simulink model "lab2"  (R2016a)
settings: Solver=VariableStepAuto  StartTime=0.0  StopTime=100  RelTol=1e-3
settings Model: Creator=ms36124  LastModifiedBy=ms36124

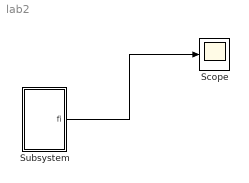
== system lab2 ==
  Scope : Scope
  Subsystem : Subsystem  mask{m=10, k=1, l=3, g=10, fi0=180}
  wires:
  Subsystem/1("fi ") -> Scope/1

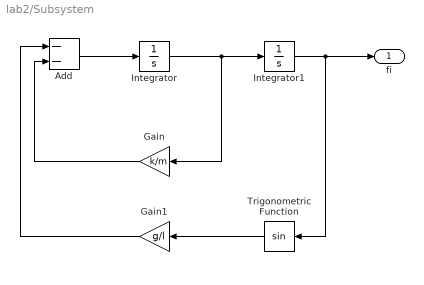
== system lab2/Subsystem ==
  Add : Sum  Inputs=--
  Gain : Gain  Gain=k/m
  Gain1 : Gain  Gain=g/l
  Integrator : Integrator
  Integrator1 : Integrator  InitialCondition=fi0*pi/180
  Trigonometric Function : Trigonometry
  "fi " : Outport
  wires:
  Trigonometric Function/1 -> Gain1/1
  Integrator/1 -> Gain/1, Integrator1/1
  Add/1 -> Integrator/1
  Integrator1/1 -> "fi "/1, Trigonometric Function/1
  Gain1/1 -> Add/1
  Gain/1 -> Add/2
